simulink model "typeAsimctrl_NB_upgrade_2016b"  (R2016b)
settings: Solver=ode45  StartTime=0.0  StopTime=12.0  RelTol=1e-3  EnableMultiTasking=on
values from neighbouring files (symbols this model uses):
  gain_actIML = 2.1e-7*1.e+6*20/(2^16)/magIM(inddc)*gain_actIML    [TypeA_reconstruction.m]
  gain_actMNL = 5.1e-6*1.e+6*20/(2^16)/magMN(inddc)*gain_actMNL    [TypeA_reconstruction.m]
  gain_actTML = 1.7e-7*1.e+6*20/(2^16)/magTM(inddc)*gain_actTML    [TypeA_reconstruction.m]
  gainBFL = 0    [main.m]
  gainIPL = 0    [main.m]
  gainSCL = 1    [TypeA_reconstruction.m]
  gainSCT = 1    [TypeA_reconstruction.m]
  sys1 = sys1_exp    [check_exportvsmake.m]    (also in sumcon2mdlconst_typeA.m = sus.ss)
undefined symbols (not defined in the file or in its folder): cMat_BF, cMat_IM, cMat_MN, cMat_TM, Filt, gain_actBFGAS, gain_actBFL, gain_actBFP, gain_actBFR, gain_actBFT, gain_actBFV, gain_actBFY, gain_actF0GAS, gain_actF1GAS, gain_actF2GAS, gain_actF3GAS, gain_actIMP, gain_actIMR, gain_actIMT, gain_actIMV, gain_actIMY, gain_actIPL, gain_actIPT, gain_actIPY, gain_actMNP, gain_actMNR, gain_actMNT, gain_actMNV, gain_actMNY, gain_actTMP, gain_actTMY, gainBFP, gainBFR, gainBFT, gainBFV, gainBFY, gainBP, gainGASBF, gainGASF0, gainGASF1, gainGASF2, gainGASF3, gainIML, gainIMP, gainIMR, gainIMT, gainIMV, gainIMY, gainIPT, gainIPY, gainLOCK_IML, gainLOCK_IMP, gainLOCK_IMY, gainMNL, gainMNLOCK_L, gainMNLOCK_P, gainMNLOCK_Y, gainMNP, gainMNR, gainMNT ... (+22)
libraries: cstblocks x77, LiveParts x77
(part 2 of 3)

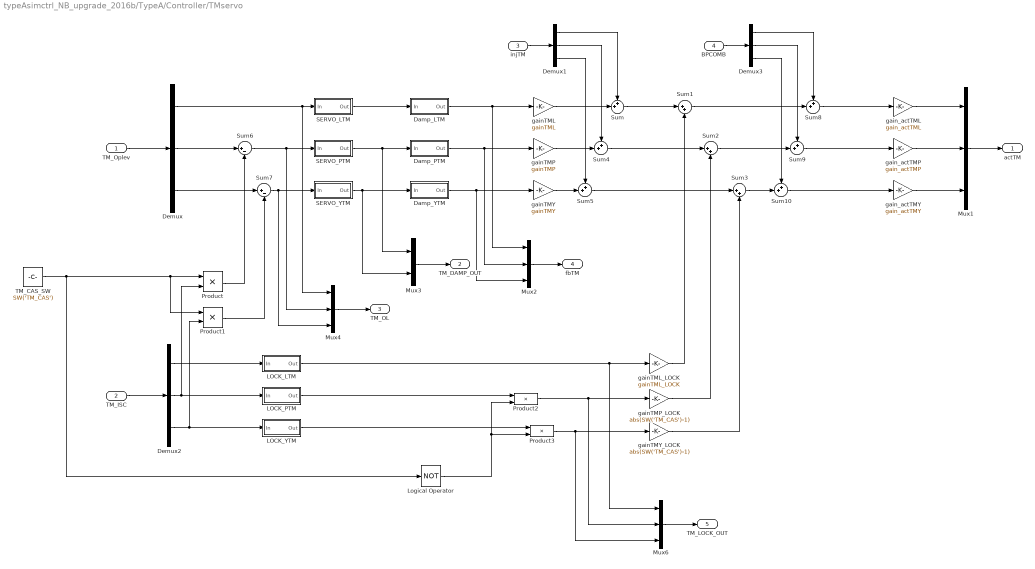
== system typeAsimctrl_NB_upgrade_2016b/TypeA/Controller/TMservo ==
  TM_Oplev : Inport
  TM_ISC : Inport  Port=2
  injTM : Inport  Port=3
  BPCOMB : Inport  Port=4
  Damp_LTM : Subsystem
  Damp_PTM : Subsystem
  Damp_YTM : Subsystem
  Demux{,1..3} (4 alike) : Demux  Outputs=3
  LOCK_LTM : Subsystem
  LOCK_PTM : Subsystem
  LOCK_YTM : Subsystem
  Logical Operator : Logic  Operator=NOT  Inputs=1  AllPortsSameDT=off  OutDataTypeStr=boolean
  Mux{1..2,4,6} (4 alike) : Mux  Inputs=3
  Mux3 : Mux  Inputs=2
  Product{,1..3} (4 alike) : Product
  SERVO_LTM : Subsystem
  SERVO_PTM : Subsystem
  SERVO_YTM : Subsystem
  Sum{,4..5,8..10} (6 alike) : Sum  Inputs=++|
  Sum1 : Sum  Inputs=|++
  Sum2 : Sum  Inputs=|++
  Sum3 : Sum  Inputs=|++
  Sum6 : Sum  Inputs=|+-
  Sum7 : Sum  Inputs=|+-
  TM_CAS_SW : Constant  Value=SW('TM_CAS')
  gainTML : Gain  Gain=gainTML
  gainTML_LOCK : Gain  Gain=gainTML_LOCK
  gainTMP : Gain  Gain=gainTMP
  gainTMP_LOCK : Gain  Gain=abs(SW('TM_CAS')-1)
  gainTMY : Gain  Gain=gainTMY
  gainTMY_LOCK : Gain  Gain=abs(SW('TM_CAS')-1)
  gain_actTML : Gain  Gain=gain_actTML
  gain_actTMP : Gain  Gain=gain_actTMP
  gain_actTMY : Gain  Gain=gain_actTMY
  actTM : Outport
  TM_DAMP_OUT : Outport  Port=2
  TM_OL : Outport  Port=3
  fbTM : Outport  Port=4
  TM_LOCK_OUT : Outport  Port=5
  wires:
  TM_Oplev/1 -> Demux/1
  gainTML/1 -> Sum/2
  injTM/1 -> Demux1/1
  Mux1/1 -> actTM/1
  Demux1/1 -> Sum/1
  gainTMP/1 -> Sum4/2
  gainTMY/1 -> Sum5/2
  gain_actTML/1 -> Mux1/1
  Demux1/2 -> Sum4/1
  Demux1/3 -> Sum5/1
  gain_actTMP/1 -> Mux1/2
  gain_actTMY/1 -> Mux1/3
  TM_ISC/1 -> Demux2/1
  SERVO_PTM/1(Out) -> Mux3/1, Damp_PTM/1(In)
  SERVO_YTM/1(Out) -> Mux3/2, Damp_YTM/1(In)
  Mux3/1 -> TM_DAMP_OUT/1
  Demux2/1 -> LOCK_LTM/1(In)
  Demux2/2 -> Product/2, LOCK_PTM/1(In)
  Demux2/3 -> Product1/2, LOCK_YTM/1(In)
  SERVO_LTM/1(Out) -> Damp_LTM/1(In)
  Sum/1 -> Sum1/1
  Sum4/1 -> Sum2/1
  Sum5/1 -> Sum3/1
  TM_CAS_SW/1 -> Logical Operator/1, Product/1, Product1/1
  Demux/2 -> Sum6/1
  Demux/3 -> Sum7/1
  Sum7/1 -> Mux4/3, SERVO_YTM/1(In)
  Product/1 -> Sum6/2
  Product1/1 -> Sum7/2
  Demux/1 -> Mux4/1, SERVO_LTM/1(In)
  Sum6/1 -> Mux4/2, SERVO_PTM/1(In)
  Mux4/1 -> TM_OL/1
  LOCK_PTM/1(Out) -> Product2/1
  Logical Operator/1 -> Product3/2, Product2/2
  LOCK_YTM/1(Out) -> Product3/1
  BPCOMB/1 -> Demux3/1
  Demux3/1 -> Sum8/1
  Demux3/2 -> Sum9/1
  Demux3/3 -> Sum10/1
  Sum1/1 -> Sum8/2
  Sum2/1 -> Sum9/2
  Sum3/1 -> Sum10/2
  Sum8/1 -> gain_actTML/1
  Sum9/1 -> gain_actTMP/1
  Sum10/1 -> gain_actTMY/1
  Damp_LTM/1(Out) -> Mux2/1, gainTML/1
  Mux2/1 -> fbTM/1
  Damp_PTM/1(Out) -> Mux2/2, gainTMP/1
  Damp_YTM/1(Out) -> Mux2/3, gainTMY/1
  Product3/1 -> Mux6/3, gainTMY_LOCK/1
  LOCK_LTM/1(Out) -> gainTML_LOCK/1, Mux6/1
  Product2/1 -> Mux6/2, gainTMP_LOCK/1
  Mux6/1 -> TM_LOCK_OUT/1
  gainTMP_LOCK/1 -> Sum2/2
  gainTML_LOCK/1 -> Sum1/2
  gainTMY_LOCK/1 -> Sum3/2

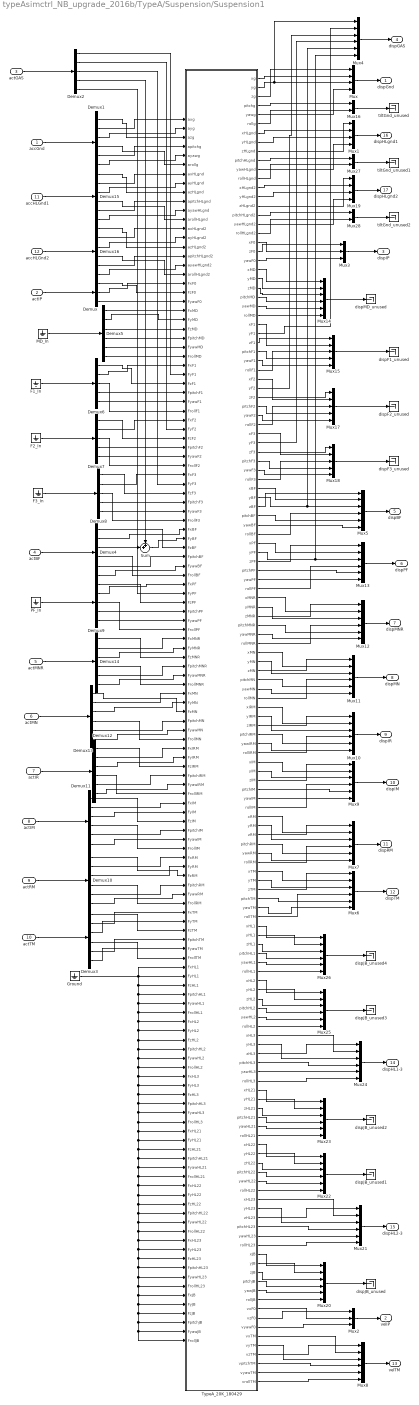
== system typeAsimctrl_NB_upgrade_2016b/TypeA/Suspension/Suspension1 ==
  accGnd : Inport
  actIP : Inport  Port=2
  actGAS : Inport  Port=3
  actBF : Inport  Port=4
  actMNR : Inport  Port=5
  actMN : Inport  Port=6
  actIR : Inport  Port=7
  actIM : Inport  Port=8
  actRM : Inport  Port=9
  actTM : Inport  Port=10
  accHLGnd1 : Inport  Port=11
  accHLGnd2 : Inport  Port=12
  Demux : Demux  Outputs=3
  Demux{1,3..5,10..16} (11 alike) : Demux  Outputs=6
  Demux{2,6..9} (5 alike) : Demux  Outputs=5
  F1_In : Ground
  F2_In : Ground
  F3_In : Ground
  Ground : Ground
  MD_In : Ground
  Mux : Mux
  Mux1 : Mux
  Mux{4..14,20..26} (18 alike) : Mux  Inputs=6
  Mux15 : Mux  Inputs=5
  Mux16 : Mux  Inputs=2
  Mux17 : Mux  Inputs=5
  Mux18 : Mux  Inputs=5
  Mux19 : Mux
  Mux2 : Mux  Inputs=3
  Mux27 : Mux  Inputs=2
  Mux28 : Mux  Inputs=2
  Mux3 : Mux  Inputs=3
  PF_In : Ground
  Sum : Sum  Inputs=++|
  TypeA_20K_180429 : Subsystem
  dispF1_unused : Terminator
  dispF2_unused : Terminator
  dispF3_unused : Terminator
  dispJB_unused{,1..4} (5 alike) : Terminator
  dispMD_unused : Terminator
  tiltGnd_unused : Terminator
  tiltGnd_unused1 : Terminator
  tiltGnd_unused2 : Terminator
  dispGnd : Outport
  velIP : Outport  Port=2
  dispIP : Outport  Port=3
  dispGAS : Outport  Port=4
  dispBF : Outport  Port=5
  dispPF : Outport  Port=6
  dispMNR : Outport  Port=7
  dispMN : Outport  Port=8
  dispIR : Outport  Port=9
  dispIM : Outport  Port=10
  dispRM : Outport  Port=11
  dispTM : Outport  Port=12
  velTM : Outport  Port=13
  dispHL1-3 : Outport  Port=14
  dispHL2-3 : Outport  Port=15
  dispHLgnd1 : Outport  Port=16
  dispHLgnd2 : Outport  Port=17
  wires:
  Mux/1 -> dispGnd/1
  Mux2/1 -> velIP/1
  Mux3/1 -> dispIP/1
  Mux4/1 -> dispGAS/1
  Mux5/1 -> dispBF/1
  Mux6/1 -> dispTM/1
  actIP/1 -> Demux/1
  accGnd/1 -> Demux1/1
  actTM/1 -> Demux3/1
  Demux4/3 -> Sum/2
  Demux2/4 -> Sum/1
  Demux2/5 -> TypeA_20K_180429/53(FyPF)
  actBF/1 -> Demux4/1
  actGAS/1 -> Demux2/1
  MD_In/1 -> Demux5/1
  Demux5/1 -> TypeA_20K_180429/22(FxMD)
  Demux5/2 -> TypeA_20K_180429/23(FyMD)
  Demux5/3 -> TypeA_20K_180429/24(FzMD)
  Demux5/4 -> TypeA_20K_180429/25(FpitchMD)
  Demux5/5 -> TypeA_20K_180429/26(FyawMD)
  Demux5/6 -> TypeA_20K_180429/27(FrollMD)
  Demux2/1 -> TypeA_20K_180429/29(FyF1)
  Demux2/2 -> TypeA_20K_180429/35(FyF2)
  Demux2/3 -> TypeA_20K_180429/41(FyF3)
  F1_In/1 -> Demux6/1
  F2_In/1 -> Demux7/1
  F3_In/1 -> Demux8/1
  Demux4/1 -> TypeA_20K_180429/48(FzBF)
  PF_In/1 -> Demux9/1
  actRM/1 -> Demux10/1
  actIM/1 -> Demux11/1
  actIR/1 -> Demux12/1
  actMN/1 -> Demux13/1
  actMNR/1 -> Demux14/1
  Demux10/5 -> TypeA_20K_180429/85(FpitchRM)
  Demux10/4 -> TypeA_20K_180429/87(FrollRM)
  Demux10/3 -> TypeA_20K_180429/83(FyRM)
  Demux10/1 -> TypeA_20K_180429/84(FzRM)
  Demux10/2 -> TypeA_20K_180429/82(FxRM)
  Demux3/3 -> TypeA_20K_180429/89(FyTM)
  Demux3/1 -> TypeA_20K_180429/90(FzTM)
  Demux3/2 -> TypeA_20K_180429/88(FxTM)
  Demux3/4 -> TypeA_20K_180429/93(FrollTM)
  Demux3/5 -> TypeA_20K_180429/91(FpitchTM)
  Demux3/6 -> TypeA_20K_180429/92(FyawTM)
  Mux7/1 -> dispRM/1
  Mux8/1 -> velTM/1
  Mux9/1 -> dispIM/1
  Mux10/1 -> dispIR/1
  Mux11/1 -> dispMN/1
  Mux12/1 -> dispMNR/1
  Mux13/1 -> dispPF/1
  Mux14/1 -> dispMD_unused/1
  Mux15/1 -> dispF1_unused/1
  Mux16/1 -> tiltGnd_unused/1
  Mux17/1 -> dispF2_unused/1
  Mux18/1 -> dispF3_unused/1
  TypeA_20K_180429/1(xg) -> Mux/2
  TypeA_20K_180429/3(zg) -> Mux/1
  TypeA_20K_180429/138(vyawF0) -> Mux2/3
  TypeA_20K_180429/19(xF0) -> Mux3/2
  TypeA_20K_180429/20(zF0) -> Mux3/1
  TypeA_20K_180429/21(yawF0) -> Mux3/3
  TypeA_20K_180429/24(zMD) -> Mux14/3
  TypeA_20K_180429/25(pitchMD) -> Mux14/4
  TypeA_20K_180429/26(yawMD) -> Mux14/5
  TypeA_20K_180429/27(rollMD) -> Mux14/6
  TypeA_20K_180429/29(yF1) -> Mux4/2
  TypeA_20K_180429/35(yF2) -> Mux4/3
  TypeA_20K_180429/41(yF3) -> Mux4/4
  TypeA_20K_180429/47(yBF) -> Mux5/3, Mux4/5
  TypeA_20K_180429/53(yPF) -> Mux13/3, Mux4/6
  TypeA_20K_180429/30(zF1) -> Mux15/1
  TypeA_20K_180429/28(xF1) -> Mux15/2
  TypeA_20K_180429/32(yawF1) -> Mux15/5
  TypeA_20K_180429/33(rollF1) -> Mux15/3
  TypeA_20K_180429/31(pitchF1) -> Mux15/4
  TypeA_20K_180429/36(zF2) -> Mux17/1
  TypeA_20K_180429/34(xF2) -> Mux17/2
  TypeA_20K_180429/39(rollF2) -> Mux17/3
  TypeA_20K_180429/38(yawF2) -> Mux17/5
  TypeA_20K_180429/37(pitchF2) -> Mux17/4
  TypeA_20K_180429/42(zF3) -> Mux18/1
  TypeA_20K_180429/40(xF3) -> Mux18/2
  TypeA_20K_180429/44(yawF3) -> Mux18/5
  TypeA_20K_180429/43(pitchF3) -> Mux18/4
  TypeA_20K_180429/45(rollF3) -> Mux18/3
  TypeA_20K_180429/49(pitchBF) -> Mux5/5
  TypeA_20K_180429/50(yawBF) -> Mux5/6
  TypeA_20K_180429/51(rollBF) -> Mux5/4
  TypeA_20K_180429/46(xBF) -> Mux5/2
  TypeA_20K_180429/48(zBF) -> Mux5/1
  TypeA_20K_180429/56(yawPF) -> Mux13/6
  TypeA_20K_180429/54(zPF) -> Mux13/1
  TypeA_20K_180429/52(xPF) -> Mux13/2
  TypeA_20K_180429/57(rollPF) -> Mux13/4
  TypeA_20K_180429/55(pitchPF) -> Mux13/5
  TypeA_20K_180429/58(xMNR) -> Mux12/2
  TypeA_20K_180429/62(yawMNR) -> Mux12/6
  TypeA_20K_180429/59(yMNR) -> Mux12/3
  TypeA_20K_180429/63(rollMNR) -> Mux12/4
  TypeA_20K_180429/60(zMNR) -> Mux12/1
  TypeA_20K_180429/61(pitchMNR) -> Mux12/5
  TypeA_20K_180429/69(rollMN) -> Mux11/4
  TypeA_20K_180429/66(zMN) -> Mux11/1
  TypeA_20K_180429/65(yMN) -> Mux11/3
  TypeA_20K_180429/64(xMN) -> Mux11/2
  TypeA_20K_180429/68(yawMN) -> Mux11/6
  TypeA_20K_180429/67(pitchMN) -> Mux11/5
  TypeA_20K_180429/73(pitchIRM) -> Mux10/5
  TypeA_20K_180429/71(yIRM) -> Mux10/3
  TypeA_20K_180429/74(yawIRM) -> Mux10/6
  TypeA_20K_180429/75(rollIRM) -> Mux10/4
  TypeA_20K_180429/70(xIRM) -> Mux10/2
  TypeA_20K_180429/72(zIRM) -> Mux10/1
  TypeA_20K_180429/78(zIM) -> Mux9/1
  TypeA_20K_180429/77(yIM) -> Mux9/3
  TypeA_20K_180429/76(xIM) -> Mux9/2
  TypeA_20K_180429/141(vzTM) -> Mux8/1
  TypeA_20K_180429/139(vxTM) -> Mux8/2
  TypeA_20K_180429/140(vyTM) -> Mux8/3
  TypeA_20K_180429/142(vpitchTM) -> Mux8/4
  TypeA_20K_180429/143(vyawTM) -> Mux8/5
  TypeA_20K_180429/144(vrollTM) -> Mux8/6
  TypeA_20K_180429/90(zTM) -> Mux6/1
  TypeA_20K_180429/88(xTM) -> Mux6/2
  TypeA_20K_180429/89(yTM) -> Mux6/3
  TypeA_20K_180429/84(zRM) -> Mux7/1
  TypeA_20K_180429/82(xRM) -> Mux7/2
  TypeA_20K_180429/83(yRM) -> Mux7/3
  TypeA_20K_180429/81(rollIM) -> Mux9/4
  TypeA_20K_180429/79(pitchIM) -> Mux9/5
  TypeA_20K_180429/80(yawIM) -> Mux9/6
  TypeA_20K_180429/87(rollRM) -> Mux7/4
  TypeA_20K_180429/85(pitchRM) -> Mux7/5
  TypeA_20K_180429/86(yawRM) -> Mux7/6
  TypeA_20K_180429/93(rollTM) -> Mux6/4
  TypeA_20K_180429/91(pitchTM) -> Mux6/5
  TypeA_20K_180429/92(yawTM) -> Mux6/6
  TypeA_20K_180429/22(xMD) -> Mux14/1
  TypeA_20K_180429/23(yMD) -> Mux14/2
  TypeA_20K_180429/136(vxF0) -> Mux2/2
  TypeA_20K_180429/137(vzF0) -> Mux2/1
  TypeA_20K_180429/2(yg) -> Mux4/1, Mux/3
  TypeA_20K_180429/5(yawg) -> Mux/4
  TypeA_20K_180429/4(pitchg) -> Mux16/1
  TypeA_20K_180429/6(rollg) -> Mux16/2
  Demux10/6 -> TypeA_20K_180429/86(FyawRM)
  Demux11/1 -> TypeA_20K_180429/78(FzIM)
  Demux11/2 -> TypeA_20K_180429/76(FxIM)
  Demux11/3 -> TypeA_20K_180429/77(FyIM)
  Demux11/4 -> TypeA_20K_180429/81(FrollIM)
  Demux11/5 -> TypeA_20K_180429/79(FpitchIM)
  Demux11/6 -> TypeA_20K_180429/80(FyawIM)
  Demux12/1 -> TypeA_20K_180429/72(FzIRM)
  Demux12/2 -> TypeA_20K_180429/70(FxIRM)
  Demux12/3 -> TypeA_20K_180429/71(FyIRM)
  Demux12/4 -> TypeA_20K_180429/75(FrollIRM)
  Demux12/5 -> TypeA_20K_180429/73(FpitchIRM)
  Demux12/6 -> TypeA_20K_180429/74(FyawIRM)
  Demux13/1 -> TypeA_20K_180429/66(FzMN)
  Demux13/2 -> TypeA_20K_180429/64(FxMN)
  Demux13/3 -> TypeA_20K_180429/65(FyMN)
  Demux13/4 -> TypeA_20K_180429/69(FrollMN)
  Demux13/5 -> TypeA_20K_180429/67(FpitchMN)
  Demux13/6 -> TypeA_20K_180429/68(FyawMN)
  Demux14/1 -> TypeA_20K_180429/60(FzMNR)
  Demux14/2 -> TypeA_20K_180429/58(FxMNR)
  Demux14/3 -> TypeA_20K_180429/59(FyMNR)
  Demux14/4 -> TypeA_20K_180429/63(FrollMNR)
  Demux14/5 -> TypeA_20K_180429/61(FpitchMNR)
  Demux14/6 -> TypeA_20K_180429/62(FyawMNR)
  Demux9/1 -> TypeA_20K_180429/54(FzPF)
  Demux9/2 -> TypeA_20K_180429/52(FxPF)
  Demux9/3 -> TypeA_20K_180429/57(FrollPF)
  Demux9/4 -> TypeA_20K_180429/55(FpitchPF)
  Demux9/5 -> TypeA_20K_180429/56(FyawPF)
  Demux4/2 -> TypeA_20K_180429/46(FxBF)
  Sum/1 -> TypeA_20K_180429/47(FyBF)
  Demux4/4 -> TypeA_20K_180429/51(FrollBF)
  Demux4/5 -> TypeA_20K_180429/49(FpitchBF)
  Demux4/6 -> TypeA_20K_180429/50(FyawBF)
  Demux8/1 -> TypeA_20K_180429/42(FzF3)
  Demux8/2 -> TypeA_20K_180429/40(FxF3)
  Demux8/3 -> TypeA_20K_180429/45(FrollF3)
  Demux8/4 -> TypeA_20K_180429/43(FpitchF3)
  Demux8/5 -> TypeA_20K_180429/44(FyawF3)
  Demux7/1 -> TypeA_20K_180429/36(FzF2)
  Demux7/2 -> TypeA_20K_180429/34(FxF2)
  Demux7/3 -> TypeA_20K_180429/39(FrollF2)
  Demux7/4 -> TypeA_20K_180429/37(FpitchF2)
  Demux7/5 -> TypeA_20K_180429/38(FyawF2)
  Demux6/1 -> TypeA_20K_180429/30(FzF1)
  Demux6/2 -> TypeA_20K_180429/28(FxF1)
  Demux6/3 -> TypeA_20K_180429/33(FrollF1)
  Demux6/4 -> TypeA_20K_180429/31(FpitchF1)
  Demux6/5 -> TypeA_20K_180429/32(FyawF1)
  Demux/1 -> TypeA_20K_180429/20(FzF0)
  Demux/2 -> TypeA_20K_180429/19(FxF0)
  Demux/3 -> TypeA_20K_180429/21(FyawF0)
  Demux1/1 -> TypeA_20K_180429/3(azg)
  Demux1/2 -> TypeA_20K_180429/1(axg)
  Demux1/3 -> TypeA_20K_180429/2(ayg)
  Demux1/4 -> TypeA_20K_180429/6(arollg)
  Demux1/5 -> TypeA_20K_180429/4(apitchg)
  Demux1/6 -> TypeA_20K_180429/5(ayawg)
  TypeA_20K_180429/132(zJB) -> Mux20/3
  TypeA_20K_180429/131(yJB) -> Mux20/2
  TypeA_20K_180429/134(yawJB) -> Mux20/5
  TypeA_20K_180429/135(rollJB) -> Mux20/6
  TypeA_20K_180429/130(xJB) -> Mux20/1
  TypeA_20K_180429/133(pitchJB) -> Mux20/4
  Mux20/1 -> dispJB_unused/1
  TypeA_20K_180429/128(yawHL23) -> Mux21/5
  TypeA_20K_180429/129(rollHL23) -> Mux21/6
  TypeA_20K_180429/124(xHL23) -> Mux21/2
  TypeA_20K_180429/127(pitchHL23) -> Mux21/4
  TypeA_20K_180429/125(yHL23) -> Mux21/3
  TypeA_20K_180429/126(zHL23) -> Mux21/1
  Mux21/1 -> dispHL2-3/1
  TypeA_20K_180429/122(yawHL22) -> Mux22/5
  TypeA_20K_180429/120(zHL22) -> Mux22/3
  TypeA_20K_180429/119(yHL22) -> Mux22/2
  TypeA_20K_180429/121(pitchHL22) -> Mux22/4
  TypeA_20K_180429/123(rollHL22) -> Mux22/6
  TypeA_20K_180429/118(xHL22) -> Mux22/1
  Mux22/1 -> dispJB_unused1/1
  TypeA_20K_180429/116(yawHL21) -> Mux23/5
  TypeA_20K_180429/114(zHL21) -> Mux23/3
  TypeA_20K_180429/113(yHL21) -> Mux23/2
  TypeA_20K_180429/115(pitchHL21) -> Mux23/4
  TypeA_20K_180429/117(rollHL21) -> Mux23/6
  TypeA_20K_180429/112(xHL21) -> Mux23/1
  Mux23/1 -> dispJB_unused2/1
  TypeA_20K_180429/110(yawHL3) -> Mux24/5
  TypeA_20K_180429/111(rollHL3) -> Mux24/6
  TypeA_20K_180429/109(pitchHL3) -> Mux24/4
  TypeA_20K_180429/107(yHL3) -> Mux24/3
  TypeA_20K_180429/108(zHL3) -> Mux24/1
  TypeA_20K_180429/106(xHL3) -> Mux24/2
  Mux24/1 -> dispHL1-3/1
  TypeA_20K_180429/104(yawHL2) -> Mux25/5
  Mux25/1 -> dispJB_unused3/1
  TypeA_20K_180429/102(zHL2) -> Mux25/3
  TypeA_20K_180429/103(pitchHL2) -> Mux25/4
  TypeA_20K_180429/105(rollHL2) -> Mux25/6
  TypeA_20K_180429/100(xHL2) -> Mux25/1
  TypeA_20K_180429/101(yHL2) -> Mux25/2
  TypeA_20K_180429/98(yawHL1) -> Mux26/5
  Mux26/1 -> dispJB_unused4/1
  TypeA_20K_180429/96(zHL1) -> Mux26/3
  TypeA_20K_180429/97(pitchHL1) -> Mux26/4
  TypeA_20K_180429/99(rollHL1) -> Mux26/6
  TypeA_20K_180429/94(xHL1) -> Mux26/1
  TypeA_20K_180429/95(yHL1) -> Mux26/2
  TypeA_20K_180429/9(zHLgnd) -> Mux1/1
  TypeA_20K_180429/7(xHLgnd) -> Mux1/2
  TypeA_20K_180429/8(yHLgnd) -> Mux1/3
  TypeA_20K_180429/11(yawHLgnd) -> Mux1/4
  Mux1/1 -> dispHLgnd1/1
  Mux19/1 -> dispHLgnd2/1
  TypeA_20K_180429/14(yHLgnd2) -> Mux19/3
  TypeA_20K_180429/15(zHLgnd2) -> Mux19/1
  TypeA_20K_180429/13(xHLgnd2) -> Mux19/2
  TypeA_20K_180429/17(yawHLgnd2) -> Mux19/4
  TypeA_20K_180429/10(pitchHLgnd) -> Mux27/1
  TypeA_20K_180429/12(rollHLgnd) -> Mux27/2
  Mux27/1 -> tiltGnd_unused1/1
  TypeA_20K_180429/16(pitchHLgnd2) -> Mux28/1
  TypeA_20K_180429/18(rollHLgnd2) -> Mux28/2
  Mux28/1 -> tiltGnd_unused2/1
  Ground/1 -> TypeA_20K_180429/96(FzHL1), TypeA_20K_180429/97(FpitchHL1), TypeA_20K_180429/98(FyawHL1), TypeA_20K_180429/99(FrollHL1), TypeA_20K_180429/100(FxHL2), TypeA_20K_180429/101(FyHL2), TypeA_20K_180429/102(FzHL2), TypeA_20K_180429/103(FpitchHL2), TypeA_20K_180429/104(FyawHL2), TypeA_20K_180429/105(FrollHL2), TypeA_20K_180429/106(FxHL3), TypeA_20K_180429/107(FyHL3), TypeA_20K_180429/108(FzHL3), TypeA_20K_180429/109(FpitchHL3), TypeA_20K_180429/110(FyawHL3), TypeA_20K_180429/111(FrollHL3), TypeA_20K_180429/112(FxHL21), TypeA_20K_180429/113(FyHL21), TypeA_20K_180429/114(FzHL21), TypeA_20K_180429/115(FpitchHL21), TypeA_20K_180429/116(FyawHL21), TypeA_20K_180429/117(FrollHL21), TypeA_20K_180429/118(FxHL22), TypeA_20K_180429/119(FyHL22), TypeA_20K_180429/120(FzHL22), TypeA_20K_180429/121(FpitchHL22), TypeA_20K_180429/122(FyawHL22), TypeA_20K_180429/123(FrollHL22), TypeA_20K_180429/124(FxHL23), TypeA_20K_180429/125(FyHL23), TypeA_20K_180429/126(FzHL23), TypeA_20K_180429/127(FpitchHL23), TypeA_20K_180429/128(FyawHL23), TypeA_20K_180429/129(FrollHL23), TypeA_20K_180429/130(FxJB), TypeA_20K_180429/131(FyJB), TypeA_20K_180429/132(FzJB), TypeA_20K_180429/133(FpitchJB), TypeA_20K_180429/134(FyawJB), TypeA_20K_180429/135(FrollJB), TypeA_20K_180429/95(FyHL1), TypeA_20K_180429/94(FxHL1)
  Demux15/4 -> TypeA_20K_180429/12(arollHLgnd)
  Demux15/5 -> TypeA_20K_180429/10(apitchHLgnd)
  Demux15/1 -> TypeA_20K_180429/9(azHLgnd)
  Demux15/2 -> TypeA_20K_180429/7(axHLgnd)
  Demux15/6 -> TypeA_20K_180429/11(ayawHLgnd)
  accHLGnd1/1 -> Demux15/1
  Demux15/3 -> TypeA_20K_180429/8(ayHLgnd)
  Demux16/4 -> TypeA_20K_180429/18(arollHLgnd2)
  Demux16/5 -> TypeA_20K_180429/16(apitchHLgnd2)
  Demux16/1 -> TypeA_20K_180429/15(azHLgnd2)
  Demux16/2 -> TypeA_20K_180429/13(axHLgnd2)
  Demux16/6 -> TypeA_20K_180429/17(ayawHLgnd2)
  accHLGnd2/1 -> Demux16/1
  Demux16/3 -> TypeA_20K_180429/14(ayHLgnd2)

== system typeAsimctrl_NB_upgrade_2016b/TypeA/Suspension/aMatrix_BF ==
  aMat_in : Inport
  cMat_BF : Constant  Value=cMat_BF  VectorParams1D=off
  coupling_BF : Product  Multiplication=Matrix(*)
  actBF : Outport
  wires:
  coupling_BF/1 -> actBF/1
  aMat_in/1 -> coupling_BF/2
  cMat_BF/1 -> coupling_BF/1

== system typeAsimctrl_NB_upgrade_2016b/TypeA/Suspension/aMatrix_GAS ==
  aMat_in : Inport
  Add{1..4} (4 alike) : Sum  Inputs=+-
  Demux4 : Demux  Outputs=5
  Mux3 : Mux  Inputs=5
  actGAS : Outport
  wires:
  aMat_in/1 -> Demux4/1
  Mux3/1 -> actGAS/1
  Add1/1 -> Mux3/1
  Add2/1 -> Mux3/2
  Demux4/3 -> Add3/1, Add2/2
  Demux4/2 -> Add1/2, Add2/1
  Demux4/1 -> Add1/1
  Demux4/5 -> Mux3/5, Add4/2
  Add4/1 -> Mux3/4
  Add3/1 -> Mux3/3
  Demux4/4 -> Add3/2, Add4/1

== system typeAsimctrl_NB_upgrade_2016b/TypeA/Suspension/aMatrix_IM ==
  aMat_in : Inport
  Gain : Gain  Gain=-1
  cMat_IM : Constant  Value=cMat_IM  VectorParams1D=off
  coupling_IM : Product  Multiplication=Matrix(*)
  actIR : Outport
  actIM : Outport  Port=2
  wires:
  coupling_IM/1 -> actIM/1, Gain/1
  aMat_in/1 -> coupling_IM/2
  cMat_IM/1 -> coupling_IM/1
  Gain/1 -> actIR/1

== system typeAsimctrl_NB_upgrade_2016b/TypeA/Suspension/aMatrix_MN ==
  aMat_in : Inport
  Gain : Gain  Gain=-1
  cMat_MN : Constant  Value=cMat_MN  VectorParams1D=off
  coupling_MN : Product  Multiplication=Matrix(*)
  actMNR : Outport
  actMN : Outport  Port=2
  wires:
  coupling_MN/1 -> actMN/1, Gain/1
  aMat_in/1 -> coupling_MN/2
  cMat_MN/1 -> coupling_MN/1
  Gain/1 -> actMNR/1

== system typeAsimctrl_NB_upgrade_2016b/TypeA/Suspension/aMatrix_TM ==
  aMat_in : Inport
  Demux : Demux  Outputs=3
  Demux1 : Demux  Outputs=3
  Gain : Gain  Gain=-1
  Ground{,1..5} (6 alike) : Ground
  Mux : Mux  Inputs=6
  Mux1 : Mux  Inputs=6
  cMat_TM : Constant  Value=cMat_TM  VectorParams1D=off
  coupling_TM : Product  Multiplication=Matrix(*)
  actRM : Outport
  actTM : Outport  Port=2
  wires:
  coupling_TM/1 -> Demux1/1, Gain/1
  aMat_in/1 -> coupling_TM/2  "3DoF"
  cMat_TM/1 -> coupling_TM/1
  Gain/1 -> Demux/1
  Demux/1 -> Mux/1
  Demux/2 -> Mux/5
  Demux/3 -> Mux/6
  Demux1/1 -> Mux1/1
  Demux1/3 -> Mux1/6
  Demux1/2 -> Mux1/5
  Ground/1 -> Mux/2
  Ground1/1 -> Mux/3
  Ground2/1 -> Mux/4
  Ground4/1 -> Mux1/3
  Ground3/1 -> Mux1/2
  Ground5/1 -> Mux1/4
  Mux/1 -> actRM/1  "6DoF"
  Mux1/1 -> actTM/1  "6DoF"

== system typeAsimctrl_NB_upgrade_2016b/TypeA/Suspension/sMatrix_BF_LVDT ==
  dispGnd : Inport
  dispBF : Inport  Port=2
  Add2 : Sum  Inputs=-+
  Demux : Demux
  Ground : Ground
  Ground1 : Ground
  Mux : Mux  Inputs=6
  BF_LVDT : Outport
  wires:
  Add2/1 -> BF_LVDT/1  "6DoF"
  dispBF/1 -> Add2/2  "6DoF"
  dispGnd/1 -> Demux/1  "4DoF"
  Demux/1 -> Mux/1  "L"
  Demux/2 -> Mux/2  "T"
  Demux/3 -> Mux/3  "V"
  Demux/4 -> Mux/6  "Y"
  Ground/1 -> Mux/4  "R"
  Ground1/1 -> Mux/5  "P"
  Mux/1 -> Add2/1

== system typeAsimctrl_NB_upgrade_2016b/TypeA/Suspension/sMatrix_GAS_LVDT ==
  dispGAS : Inport
  Add{1..5} (5 alike) : Sum  Inputs=-+
  Demux4 : Demux  Outputs=6
  Mux3 : Mux  Inputs=5
  GAS_LVDT : Outport
  wires:
  dispGAS/1 -> Demux4/1
  Demux4/1 -> Add2/1  "VGnd = IPV"
  Demux4/2 -> Add1/1, Add2/2  "VF1"
  Demux4/3 -> Add1/2, Add3/1  "VF2"
  Demux4/4 -> Add4/1, Add3/2  "VF3"
  Add2/1 -> Mux3/1  "GASF0"
  Add1/1 -> Mux3/2  "GASF1"
  Add3/1 -> Mux3/3  "GASF2"
  Mux3/1 -> GAS_LVDT/1
  Demux4/5 -> Add5/1, Add4/2  "VBF"
  Demux4/6 -> Add5/2  "VPF"
  Add4/1 -> Mux3/4  "GASF3"
  Add5/1 -> Mux3/5  "GASBF"

== system typeAsimctrl_NB_upgrade_2016b/TypeA/Suspension/sMatrix_IM_PS ==
  dispIR : Inport
  dispIM : Inport  Port=2
  Add2 : Sum  Inputs=-+
  IM_PS : Outport
  wires:
  Add2/1 -> IM_PS/1
  dispIM/1 -> Add2/2
  dispIR/1 -> Add2/1

== system typeAsimctrl_NB_upgrade_2016b/TypeA/Suspension/sMatrix_IP_LVDT ==
  dispGnd : Inport
  dispIP : Inport  Port=2
  Add2 : Sum  Inputs=-+
  Demux : Demux
  Mux : Mux  Inputs=3
  Terminator : Terminator
  IP_LVDT : Outport
  wires:
  Add2/1 -> IP_LVDT/1
  dispIP/1 -> Add2/2
  dispGnd/1 -> Demux/1
  Demux/1 -> Mux/1  "L"
  Demux/2 -> Mux/2  "T"
  Demux/4 -> Mux/3  "Y"
  Demux/3 -> Terminator/1  "V"
  Mux/1 -> Add2/1

== system typeAsimctrl_NB_upgrade_2016b/TypeA/Suspension/sMatrix_MN_OpLev ==
  dispMN : Inport
  dispGND : Inport  Port=2
  Demux : Demux  Outputs=6
  Demux1 : Demux
  Mux : Mux  Inputs=6
  Sum : Sum  Inputs=-+|
  Sum1 : Sum  Inputs=-+|
  Sum2 : Sum  Inputs=-+|
  Terminator : Terminator
  MN_OpLev : Outport
  wires:
  dispMN/1 -> Demux/1
  dispGND/1 -> Demux1/1
  Demux/1 -> Sum/2
  Demux1/1 -> Sum/1
  Demux1/2 -> Sum1/1
  Demux/2 -> Sum1/2
  Demux/3 -> Sum2/2
  Demux1/3 -> Sum2/1
  Demux1/4 -> Terminator/1
  Sum/1 -> Mux/1
  Sum1/1 -> Mux/2
  Sum2/1 -> Mux/3
  Demux/4 -> Mux/4
  Demux/5 -> Mux/5
  Demux/6 -> Mux/6
  Mux/1 -> MN_OpLev/1

== system typeAsimctrl_NB_upgrade_2016b/TypeA/Suspension/sMatrix_MN_PS ==
  dispMNR : Inport
  dispMN : Inport  Port=2
  Add2 : Sum  Inputs=-+
  MN_PS : Outport
  wires:
  Add2/1 -> MN_PS/1
  dispMN/1 -> Add2/2
  dispMNR/1 -> Add2/1

== system typeAsimctrl_NB_upgrade_2016b/TypeA/Suspension/sMatrix_PF_OpLev ==
  dispPF : Inport
  dispGND : Inport  Port=2
  Demux : Demux
  Demux4 : Demux  Outputs=6
  Mux3 : Mux  Inputs=3
  Sum : Sum  Inputs=-+|
  Terminator : Terminator
  Terminator1 : Terminator
  Terminator2 : Terminator
  dispRPF : Terminator
  dispTPF : Terminator
  dispVPF : Terminator
  OpLev_PF : Outport
  wires:
  dispPF/1 -> Demux4/1
  Mux3/1 -> OpLev_PF/1
  Demux4/2 -> dispTPF/1
  Demux4/3 -> dispVPF/1
  Demux4/5 -> Mux3/2
  Demux4/6 -> Mux3/3
  Demux4/4 -> dispRPF/1
  Demux4/1 -> Sum/2
  Sum/1 -> Mux3/1
  dispGND/1 -> Demux/1
  Demux/1 -> Sum/1
  Demux/2 -> Terminator/1
  Demux/3 -> Terminator1/1
  Demux/4 -> Terminator2/1

== system typeAsimctrl_NB_upgrade_2016b/TypeA/Suspension/sMatrix_TM_OpLev ==
  dispTM : Inport
  dispGND : Inport  Port=2
  Add : Sum  Inputs=-+
  Demux : Demux
  Demux4 : Demux  Outputs=6
  Mux3 : Mux  Inputs=3
  dispTMR : Terminator
  dispTMT{,1..3} (4 alike) : Terminator
  dispTMV : Terminator
  TM_OpLev : Outport
  wires:
  dispTM/1 -> Demux4/1
  Mux3/1 -> TM_OpLev/1
  Demux4/2 -> dispTMT/1
  Demux4/3 -> dispTMV/1
  Demux4/4 -> dispTMR/1
  Demux4/5 -> Mux3/2
  Demux4/6 -> Mux3/3
  Demux/1 -> Add/1
  dispGND/1 -> Demux/1
  Demux/2 -> dispTMT1/1
  Demux/3 -> dispTMT2/1
  Demux/4 -> dispTMT3/1
  Demux4/1 -> Add/2
  Add/1 -> Mux3/1

== system typeAsimctrl_NB_upgrade_2016b/TypeA/Suspension/sMatrix_TM_PS ==
  dispRM : Inport
  dispTM : Inport  Port=2
  Add2 : Sum  Inputs=-+
  Demux : Demux  Outputs=6
  Demux1 : Demux  Outputs=6
  Mux : Mux  Inputs=3
  Mux1 : Mux  Inputs=3
  Terminator{,1..5} (6 alike) : Terminator
  TM_PS : Outport
  wires:
  Add2/1 -> TM_PS/1  "(L, P, Y)"
  dispRM/1 -> Demux/1
  dispTM/1 -> Demux1/1
  Demux/1 -> Mux/1  "L"
  Demux/5 -> Mux/2  "P"
  Demux/6 -> Mux/3  "Y"
  Demux1/1 -> Mux1/1  "L"
  Demux1/5 -> Mux1/2  "P"
  Demux1/6 -> Mux1/3  "Y"
  Mux/1 -> Add2/1
  Mux1/1 -> Add2/2
  Demux/2 -> Terminator/1  "T"
  Demux/4 -> Terminator2/1  "R"
  Demux/3 -> Terminator1/1  "V"
  Demux1/4 -> Terminator5/1  "R"
  Demux1/2 -> Terminator3/1  "T"
  Demux1/3 -> Terminator4/1  "V"

== system typeAsimctrl_NB_upgrade_2016b/TypeA/Controller/BFservo/Servo_LBF ==
  In : Inport
  BF_DAMP_L : cstblocks/LTI System  sys=Filt('BF_DAMP_L')  IC=[]
  K1:VIS-OPTIC_BF_DAMP_L : LiveParts/LiveFilter  Tag=LiveFilter
      settings: AttributesFormatString=%<Tag>
  Out : Outport
  wires:
  In/1 -> BF_DAMP_L/1
  BF_DAMP_L/1 -> Out/1

== system typeAsimctrl_NB_upgrade_2016b/TypeA/Controller/BFservo/Servo_PBF ==
  In : Inport
  BF_DAMP_P : cstblocks/LTI System  sys=Filt('BF_DAMP_P')  IC=[]
  K1:VIS-OPTIC_BF_DAMP_P : LiveParts/LiveFilter  Tag=LiveFilter
      settings: AttributesFormatString=%<Tag>
  Out : Outport
  wires:
  In/1 -> BF_DAMP_P/1
  BF_DAMP_P/1 -> Out/1

== system typeAsimctrl_NB_upgrade_2016b/TypeA/Controller/BFservo/Servo_RBF ==
  In : Inport
  BF_DAMP_R : cstblocks/LTI System  sys=Filt('BF_DAMP_R')  IC=[]
  K1:VIS-OPTIC_BF_DAMP_R : LiveParts/LiveFilter  Tag=LiveFilter
      settings: AttributesFormatString=%<Tag>
  Out : Outport
  wires:
  In/1 -> BF_DAMP_R/1
  BF_DAMP_R/1 -> Out/1

== system typeAsimctrl_NB_upgrade_2016b/TypeA/Controller/BFservo/Servo_TBF ==
  In : Inport
  BF_DAMP_T : cstblocks/LTI System  sys=Filt('BF_DAMP_T')  IC=[]
  K1:VIS-OPTIC_BF_DAMP_T : LiveParts/LiveFilter  Tag=LiveFilter
      settings: AttributesFormatString=%<Tag>
  Out : Outport
  wires:
  In/1 -> BF_DAMP_T/1
  BF_DAMP_T/1 -> Out/1

== system typeAsimctrl_NB_upgrade_2016b/TypeA/Controller/BFservo/Servo_VBF ==
  In : Inport
  BF_DAMP_V : cstblocks/LTI System  sys=Filt('BF_DAMP_V')  IC=[]
  K1:VIS-OPTIC_BF_DAMP_V : LiveParts/LiveFilter  Tag=LiveFilter
      settings: AttributesFormatString=%<Tag>
  Out : Outport
  wires:
  In/1 -> BF_DAMP_V/1
  BF_DAMP_V/1 -> Out/1

== system typeAsimctrl_NB_upgrade_2016b/TypeA/Controller/BFservo/Servo_YBF ==
  In : Inport
  BF_DAMP_Y : cstblocks/LTI System  sys=Filt('BF_DAMP_Y')  IC=[]
  K1:VIS-OPTIC_BF_DAMP_Y : LiveParts/LiveFilter  Tag=LiveFilter
      settings: AttributesFormatString=%<Tag>
  Out : Outport
  wires:
  In/1 -> BF_DAMP_Y/1
  BF_DAMP_Y/1 -> Out/1

== system typeAsimctrl_NB_upgrade_2016b/TypeA/Controller/BPcomb/OLSERVO_20 ==
  In : Inport
  K1:VIS-OPTIC_PAY_OLSERVO_DAMP_P20 : LiveParts/LiveFilter  Tag=LiveFilter
      settings: AttributesFormatString=%<Tag>
  PAY_OLSERVO_DAMP_P20 : cstblocks/LTI System  sys=Filt('PAY_OLSERVO_DAMP_P20')  IC=[]
  Out : Outport
  wires:
  In/1 -> PAY_OLSERVO_DAMP_P20/1
  PAY_OLSERVO_DAMP_P20/1 -> Out/1

== system typeAsimctrl_NB_upgrade_2016b/TypeA/Controller/BPcomb/OLSERVO_22 ==
  In : Inport
  K1:VIS-OPTIC_PAY_OLSERVO_DAMP_P22 : LiveParts/LiveFilter  Tag=LiveFilter
      settings: AttributesFormatString=%<Tag>
  PAY_OLSERVO_DAMP_P22 : cstblocks/LTI System  sys=Filt('PAY_OLSERVO_DAMP_P22')  IC=[]
  Out : Outport
  wires:
  In/1 -> PAY_OLSERVO_DAMP_P22/1
  PAY_OLSERVO_DAMP_P22/1 -> Out/1

== system typeAsimctrl_NB_upgrade_2016b/TypeA/Controller/BPcomb/OLSERVO_P01 ==
  In : Inport
  K1:VIS-OPTIC_PAY_OLSERVO_DAMP_P01 : LiveParts/LiveFilter  Tag=LiveFilter
      settings: AttributesFormatString=%<Tag>
  PAY_OLSERVO_DAMP_P01 : cstblocks/LTI System  sys=Filt('PAY_OLSERVO_DAMP_P01')  IC=[]
  Out : Outport
  wires:
  In/1 -> PAY_OLSERVO_DAMP_P01/1
  PAY_OLSERVO_DAMP_P01/1 -> Out/1

== system typeAsimctrl_NB_upgrade_2016b/TypeA/Controller/BPcomb/OLSERVO_P02 ==
  In : Inport
  K1:VIS-OPTIC_PAY_OLSERVO_DAMP_P02 : LiveParts/LiveFilter  Tag=LiveFilter
      settings: AttributesFormatString=%<Tag>
  PAY_OLSERVO_DAMP_P02 : cstblocks/LTI System  sys=Filt('PAY_OLSERVO_DAMP_P02')  IC=[]
  Out : Outport
  wires:
  In/1 -> PAY_OLSERVO_DAMP_P02/1
  PAY_OLSERVO_DAMP_P02/1 -> Out/1

== system typeAsimctrl_NB_upgrade_2016b/TypeA/Controller/BPcomb/OLSERVO_P03 ==
  In : Inport
  K1:VIS-OPTIC_PAY_OLSERVO_DAMP_P03 : LiveParts/LiveFilter  Tag=LiveFilter
      settings: AttributesFormatString=%<Tag>
  PAY_OLSERVO_DAMP_P03 : cstblocks/LTI System  sys=Filt('PAY_OLSERVO_DAMP_P03')  IC=[]
  Out : Outport
  wires:
  In/1 -> PAY_OLSERVO_DAMP_P03/1
  PAY_OLSERVO_DAMP_P03/1 -> Out/1

== system typeAsimctrl_NB_upgrade_2016b/TypeA/Controller/BPcomb/OLSERVO_P04 ==
  In : Inport
  K1:VIS-OPTIC_PAY_OLSERVO_DAMP_P04 : LiveParts/LiveFilter  Tag=LiveFilter
      settings: AttributesFormatString=%<Tag>
  PAY_OLSERVO_DAMP_P04 : cstblocks/LTI System  sys=Filt('PAY_OLSERVO_DAMP_P04')  IC=[]
  Out : Outport
  wires:
  In/1 -> PAY_OLSERVO_DAMP_P04/1
  PAY_OLSERVO_DAMP_P04/1 -> Out/1

== system typeAsimctrl_NB_upgrade_2016b/TypeA/Controller/BPcomb/OLSERVO_P05 ==
  In : Inport
  K1:VIS-OPTIC_PAY_OLSERVO_DAMP_P05 : LiveParts/LiveFilter  Tag=LiveFilter
      settings: AttributesFormatString=%<Tag>
  PAY_OLSERVO_DAMP_P05 : cstblocks/LTI System  sys=Filt('PAY_OLSERVO_DAMP_P05')  IC=[]
  Out : Outport
  wires:
  In/1 -> PAY_OLSERVO_DAMP_P05/1
  PAY_OLSERVO_DAMP_P05/1 -> Out/1

== system typeAsimctrl_NB_upgrade_2016b/TypeA/Controller/BPcomb/OLSERVO_P06 ==
  In : Inport
  K1:VIS-OPTIC_PAY_OLSERVO_DAMP_P06 : LiveParts/LiveFilter  Tag=LiveFilter
      settings: AttributesFormatString=%<Tag>
  PAY_OLSERVO_DAMP_P06 : cstblocks/LTI System  sys=Filt('PAY_OLSERVO_DAMP_P06')  IC=[]
  Out : Outport
  wires:
  In/1 -> PAY_OLSERVO_DAMP_P06/1
  PAY_OLSERVO_DAMP_P06/1 -> Out/1

== system typeAsimctrl_NB_upgrade_2016b/TypeA/Controller/BPcomb/OLSERVO_P07 ==
  In : Inport
  K1:VIS-OPTIC_PAY_OLSERVO_DAMP_P07 : LiveParts/LiveFilter  Tag=LiveFilter
      settings: AttributesFormatString=%<Tag>
  PAY_OLSERVO_DAMP_P07 : cstblocks/LTI System  sys=Filt('PAY_OLSERVO_DAMP_P07')  IC=[]
  Out : Outport
  wires:
  In/1 -> PAY_OLSERVO_DAMP_P07/1
  PAY_OLSERVO_DAMP_P07/1 -> Out/1

== system typeAsimctrl_NB_upgrade_2016b/TypeA/Controller/BPcomb/OLSERVO_P08 ==
  In : Inport
  K1:VIS-OPTIC_PAY_OLSERVO_DAMP_P08 : LiveParts/LiveFilter  Tag=LiveFilter
      settings: AttributesFormatString=%<Tag>
  PAY_OLSERVO_DAMP_P08 : cstblocks/LTI System  sys=Filt('PAY_OLSERVO_DAMP_P08')  IC=[]
  Out : Outport
  wires:
  In/1 -> PAY_OLSERVO_DAMP_P08/1
  PAY_OLSERVO_DAMP_P08/1 -> Out/1

== system typeAsimctrl_NB_upgrade_2016b/TypeA/Controller/BPcomb/OLSERVO_P09 ==
  In : Inport
  K1:VIS-OPTIC_PAY_OLSERVO_DAMP_P09 : LiveParts/LiveFilter  Tag=LiveFilter
      settings: AttributesFormatString=%<Tag>
  PAY_OLSERVO_DAMP_P09 : cstblocks/LTI System  sys=Filt('PAY_OLSERVO_DAMP_P09')  IC=[]
  Out : Outport
  wires:
  In/1 -> PAY_OLSERVO_DAMP_P09/1
  PAY_OLSERVO_DAMP_P09/1 -> Out/1

== system typeAsimctrl_NB_upgrade_2016b/TypeA/Controller/BPcomb/OLSERVO_P10 ==
  In : Inport
  K1:VIS-OPTIC_PAY_OLSERVO_DAMP_P10 : LiveParts/LiveFilter  Tag=LiveFilter
      settings: AttributesFormatString=%<Tag>
  PAY_OLSERVO_DAMP_P10 : cstblocks/LTI System  sys=Filt('PAY_OLSERVO_DAMP_P10')  IC=[]
  Out : Outport
  wires:
  In/1 -> PAY_OLSERVO_DAMP_P10/1
  PAY_OLSERVO_DAMP_P10/1 -> Out/1

== system typeAsimctrl_NB_upgrade_2016b/TypeA/Controller/BPcomb/OLSERVO_P11 ==
  In : Inport
  K1:VIS-OPTIC_PAY_OLSERVO_DAMP_P11 : LiveParts/LiveFilter  Tag=LiveFilter
      settings: AttributesFormatString=%<Tag>
  PAY_OLSERVO_DAMP_P11 : cstblocks/LTI System  sys=Filt('PAY_OLSERVO_DAMP_P11')  IC=[]
  Out : Outport
  wires:
  In/1 -> PAY_OLSERVO_DAMP_P11/1
  PAY_OLSERVO_DAMP_P11/1 -> Out/1

== system typeAsimctrl_NB_upgrade_2016b/TypeA/Controller/BPcomb/OLSERVO_P12 ==
  In : Inport
  K1:VIS-OPTIC_PAY_OLSERVO_DAMP_P12 : LiveParts/LiveFilter  Tag=LiveFilter
      settings: AttributesFormatString=%<Tag>
  PAY_OLSERVO_DAMP_P12 : cstblocks/LTI System  sys=Filt('PAY_OLSERVO_DAMP_P12')  IC=[]
  Out : Outport
  wires:
  In/1 -> PAY_OLSERVO_DAMP_P12/1
  PAY_OLSERVO_DAMP_P12/1 -> Out/1

== system typeAsimctrl_NB_upgrade_2016b/TypeA/Controller/BPcomb/OLSERVO_P13 ==
  In : Inport
  K1:VIS-OPTIC_PAY_OLSERVO_DAMP_P13 : LiveParts/LiveFilter  Tag=LiveFilter
      settings: AttributesFormatString=%<Tag>
  PAY_OLSERVO_DAMP_P13 : cstblocks/LTI System  sys=Filt('PAY_OLSERVO_DAMP_P13')  IC=[]
  Out : Outport
  wires:
  In/1 -> PAY_OLSERVO_DAMP_P13/1
  PAY_OLSERVO_DAMP_P13/1 -> Out/1

== system typeAsimctrl_NB_upgrade_2016b/TypeA/Controller/BPcomb/OLSERVO_P14 ==
  In : Inport
  K1:VIS-OPTIC_PAY_OLSERVO_DAMP_P14 : LiveParts/LiveFilter  Tag=LiveFilter
      settings: AttributesFormatString=%<Tag>
  PAY_OLSERVO_DAMP_P14 : cstblocks/LTI System  sys=Filt('PAY_OLSERVO_DAMP_P14')  IC=[]
  Out : Outport
  wires:
  In/1 -> PAY_OLSERVO_DAMP_P14/1
  PAY_OLSERVO_DAMP_P14/1 -> Out/1

== system typeAsimctrl_NB_upgrade_2016b/TypeA/Controller/BPcomb/OLSERVO_P15 ==
  In : Inport
  K1:VIS-OPTIC_PAY_OLSERVO_DAMP_P15 : LiveParts/LiveFilter  Tag=LiveFilter
      settings: AttributesFormatString=%<Tag>
  PAY_OLSERVO_DAMP_P15 : cstblocks/LTI System  sys=Filt('PAY_OLSERVO_DAMP_P15')  IC=[]
  Out : Outport
  wires:
  In/1 -> PAY_OLSERVO_DAMP_P15/1
  PAY_OLSERVO_DAMP_P15/1 -> Out/1

== system typeAsimctrl_NB_upgrade_2016b/TypeA/Controller/BPcomb/OLSERVO_P16 ==
  In : Inport
  K1:VIS-OPTIC_PAY_OLSERVO_DAMP_P16 : LiveParts/LiveFilter  Tag=LiveFilter
      settings: AttributesFormatString=%<Tag>
  PAY_OLSERVO_DAMP_P16 : cstblocks/LTI System  sys=Filt('PAY_OLSERVO_DAMP_P16')  IC=[]
  Out : Outport
  wires:
  In/1 -> PAY_OLSERVO_DAMP_P16/1
  PAY_OLSERVO_DAMP_P16/1 -> Out/1

== system typeAsimctrl_NB_upgrade_2016b/TypeA/Controller/BPcomb/OLSERVO_P17 ==
  In : Inport
  K1:VIS-OPTIC_PAY_OLSERVO_DAMP_P17 : LiveParts/LiveFilter  Tag=LiveFilter
      settings: AttributesFormatString=%<Tag>
  PAY_OLSERVO_DAMP_P17 : cstblocks/LTI System  sys=Filt('PAY_OLSERVO_DAMP_P17')  IC=[]
  Out : Outport
  wires:
  In/1 -> PAY_OLSERVO_DAMP_P17/1
  PAY_OLSERVO_DAMP_P17/1 -> Out/1

== system typeAsimctrl_NB_upgrade_2016b/TypeA/Controller/BPcomb/OLSERVO_P18 ==
  In : Inport
  K1:VIS-OPTIC_PAY_OLSERVO_DAMP_P18 : LiveParts/LiveFilter  Tag=LiveFilter
      settings: AttributesFormatString=%<Tag>
  PAY_OLSERVO_DAMP_P18 : cstblocks/LTI System  sys=Filt('PAY_OLSERVO_DAMP_P18')  IC=[]
  Out : Outport
  wires:
  In/1 -> PAY_OLSERVO_DAMP_P18/1
  PAY_OLSERVO_DAMP_P18/1 -> Out/1

== system typeAsimctrl_NB_upgrade_2016b/TypeA/Controller/BPcomb/OLSERVO_P19 ==
  In : Inport
  K1:VIS-OPTIC_PAY_OLSERVO_DAMP_P19 : LiveParts/LiveFilter  Tag=LiveFilter
      settings: AttributesFormatString=%<Tag>
  PAY_OLSERVO_DAMP_P19 : cstblocks/LTI System  sys=Filt('PAY_OLSERVO_DAMP_P19')  IC=[]
  Out : Outport
  wires:
  In/1 -> PAY_OLSERVO_DAMP_P19/1
  PAY_OLSERVO_DAMP_P19/1 -> Out/1

== system typeAsimctrl_NB_upgrade_2016b/TypeA/Controller/BPcomb/OLSERVO_P21 ==
  In : Inport
  K1:VIS-OPTIC_PAY_OLSERVO_DAMP_P07 : LiveParts/LiveFilter  Tag=LiveFilter
      settings: AttributesFormatString=%<Tag>
  PAY_OLSERVO_DAMP_P21 : cstblocks/LTI System  sys=Filt('PAY_OLSERVO_DAMP_P21')  IC=[]
  Out : Outport
  wires:
  In/1 -> PAY_OLSERVO_DAMP_P21/1
  PAY_OLSERVO_DAMP_P21/1 -> Out/1

== system typeAsimctrl_NB_upgrade_2016b/TypeA/Controller/BPcomb/OLSERVO_P23 ==
  In : Inport
  K1:VIS-OPTIC_PAY_OLSERVO_DAMP_P23 : LiveParts/LiveFilter  Tag=LiveFilter
      settings: AttributesFormatString=%<Tag>
  PAY_OLSERVO_DAMP_P23 : cstblocks/LTI System  sys=Filt('PAY_OLSERVO_DAMP_P23')  IC=[]
  Out : Outport
  wires:
  In/1 -> PAY_OLSERVO_DAMP_P23/1
  PAY_OLSERVO_DAMP_P23/1 -> Out/1

== system typeAsimctrl_NB_upgrade_2016b/TypeA/Controller/BPcomb/OLSERVO_P24 ==
  In : Inport
  K1:VIS-OPTIC_PAY_OLSERVO_DAMP_P24 : LiveParts/LiveFilter  Tag=LiveFilter
      settings: AttributesFormatString=%<Tag>
  PAY_OLSERVO_DAMP_P24 : cstblocks/LTI System  sys=Filt('PAY_OLSERVO_DAMP_P24')  IC=[]
  Out : Outport
  wires:
  In/1 -> PAY_OLSERVO_DAMP_P24/1
  PAY_OLSERVO_DAMP_P24/1 -> Out/1

== system typeAsimctrl_NB_upgrade_2016b/TypeA/Controller/GASservo/Servo_GASBF ==
  In : Inport
  BF_DAMP_GAS : cstblocks/LTI System  sys=Filt('BF_DAMP_GAS')  IC=[]
  K1:VIS-OPTIC_BF_DAMP_GAS : LiveParts/LiveFilter  Tag=LiveFilter
      settings: AttributesFormatString=%<Tag>
  Out : Outport
  wires:
  In/1 -> BF_DAMP_GAS/1
  BF_DAMP_GAS/1 -> Out/1

== system typeAsimctrl_NB_upgrade_2016b/TypeA/Controller/GASservo/Servo_GASF0 ==
  In : Inport
  F0_DAMP_GAS : cstblocks/LTI System  sys=Filt('F0_DAMP_GAS')  IC=[]
  K1:VIS-OPTIC_F0_DAMP_GAS : LiveParts/LiveFilter  Tag=LiveFilter
      settings: AttributesFormatString=%<Tag>
  Out : Outport
  wires:
  In/1 -> F0_DAMP_GAS/1
  F0_DAMP_GAS/1 -> Out/1

== system typeAsimctrl_NB_upgrade_2016b/TypeA/Controller/GASservo/Servo_GASF1 ==
  In : Inport
  F1_DAMP_GAS : cstblocks/LTI System  sys=Filt('F1_DAMP_GAS')  IC=[]
  K1:VIS-OPTIC_F1_DAMP_GAS : LiveParts/LiveFilter  Tag=LiveFilter
      settings: AttributesFormatString=%<Tag>
  Out : Outport
  wires:
  In/1 -> F1_DAMP_GAS/1
  F1_DAMP_GAS/1 -> Out/1

== system typeAsimctrl_NB_upgrade_2016b/TypeA/Controller/GASservo/Servo_GASF2 ==
  In : Inport
  F2_DAMP_GAS : cstblocks/LTI System  sys=Filt('F2_DAMP_GAS')  IC=[]
  K1:VIS-OPTIC_F2_DAMP_GAS : LiveParts/LiveFilter  Tag=LiveFilter
      settings: AttributesFormatString=%<Tag>
  Out : Outport
  wires:
  In/1 -> F2_DAMP_GAS/1
  F2_DAMP_GAS/1 -> Out/1

== system typeAsimctrl_NB_upgrade_2016b/TypeA/Controller/GASservo/Servo_GASF3 ==
  In : Inport
  F3_DAMP_GAS : cstblocks/LTI System  sys=Filt('F3_DAMP_GAS')  IC=[]
  K1:VIS-OPTIC_F3_DAMP_GAS : LiveParts/LiveFilter  Tag=LiveFilter
      settings: AttributesFormatString=%<Tag>
  Out : Outport
  wires:
  In/1 -> F3_DAMP_GAS/1
  F3_DAMP_GAS/1 -> Out/1

== system typeAsimctrl_NB_upgrade_2016b/TypeA/Controller/IMservo/Damp_LIM ==
  In : Inport
  IM_PSDAMP_L : cstblocks/LTI System  sys=Filt('IM_PSDAMP_L')  IC=[]
  K1:VIS-OPTIC_IM_PSDAMP_L : LiveParts/LiveFilter  Tag=LiveFilter
      settings: AttributesFormatString=%<Tag>
  Out : Outport
  wires:
  In/1 -> IM_PSDAMP_L/1
  IM_PSDAMP_L/1 -> Out/1

== system typeAsimctrl_NB_upgrade_2016b/TypeA/Controller/IMservo/Damp_PIM ==
  In : Inport
  IM_PSDAMP_P : cstblocks/LTI System  sys=Filt('IM_PSDAMP_P')  IC=[]
  K1:VIS-OPTIC_IM_PSDAMP_P : LiveParts/LiveFilter  Tag=LiveFilter
      settings: AttributesFormatString=%<Tag>
  Out : Outport
  wires:
  In/1 -> IM_PSDAMP_P/1
  IM_PSDAMP_P/1 -> Out/1

== system typeAsimctrl_NB_upgrade_2016b/TypeA/Controller/IMservo/Damp_RIM ==
  In : Inport
  IM_PSDAMP_R : cstblocks/LTI System  sys=Filt('IM_PSDAMP_R')  IC=[]
  K1:VIS-OPTIC_IM_PSDAMP_R : LiveParts/LiveFilter  Tag=LiveFilter
      settings: AttributesFormatString=%<Tag>
  Out : Outport
  wires:
  In/1 -> IM_PSDAMP_R/1
  IM_PSDAMP_R/1 -> Out/1

== system typeAsimctrl_NB_upgrade_2016b/TypeA/Controller/IMservo/Damp_TIM ==
  In : Inport
  IM_PSDAMP_T : cstblocks/LTI System  sys=Filt('IM_PSDAMP_T')  IC=[]
  K1:VIS-OPTIC_IM_PSDAMP_T : LiveParts/LiveFilter  Tag=LiveFilter
      settings: AttributesFormatString=%<Tag>
  Out : Outport
  wires:
  In/1 -> IM_PSDAMP_T/1
  IM_PSDAMP_T/1 -> Out/1

== system typeAsimctrl_NB_upgrade_2016b/TypeA/Controller/IMservo/Damp_VIM ==
  In : Inport
  IM_PSDAMP_V : cstblocks/LTI System  sys=Filt('IM_PSDAMP_V')  IC=[]
  K1:VIS-OPTIC_IM_PSDAMP_V : LiveParts/LiveFilter  Tag=LiveFilter
      settings: AttributesFormatString=%<Tag>
  Out : Outport
  wires:
  In/1 -> IM_PSDAMP_V/1
  IM_PSDAMP_V/1 -> Out/1

== system typeAsimctrl_NB_upgrade_2016b/TypeA/Controller/IMservo/Damp_YIM ==
  In : Inport
  IM_PSDAMP_Y : cstblocks/LTI System  sys=Filt('IM_PSDAMP_Y')  IC=[]
  K1:VIS-OPTIC_IM_PSDAMP_Y : LiveParts/LiveFilter  Tag=LiveFilter
      settings: AttributesFormatString=%<Tag>
  Out : Outport
  wires:
  In/1 -> IM_PSDAMP_Y/1
  IM_PSDAMP_Y/1 -> Out/1

== system typeAsimctrl_NB_upgrade_2016b/TypeA/Controller/IMservo/IMLOCK_L ==
  In : Inport
  IM_LOCK_L : cstblocks/LTI System  sys=Filt('IM_LOCK_L')  IC=[]
  K1:VIS-OPTIC_IM_LOCK_L : LiveParts/LiveFilter  Tag=LiveFilter
      settings: AttributesFormatString=%<Tag>
  Out : Outport
  wires:
  In/1 -> IM_LOCK_L/1
  IM_LOCK_L/1 -> Out/1

== system typeAsimctrl_NB_upgrade_2016b/TypeA/Controller/IMservo/IMLOCK_P ==
  In : Inport
  IM_LOCK_P : cstblocks/LTI System  sys=Filt('IM_LOCK_P')  IC=[]
  K1:VIS-OPTIC_IM_LOCK_P : LiveParts/LiveFilter  Tag=LiveFilter
      settings: AttributesFormatString=%<Tag>
  Out : Outport
  wires:
  In/1 -> IM_LOCK_P/1
  IM_LOCK_P/1 -> Out/1

== system typeAsimctrl_NB_upgrade_2016b/TypeA/Controller/IMservo/IMLOCK_Y ==
  In : Inport
  IM_LOCK_Y : cstblocks/LTI System  sys=Filt('IM_LOCK_Y')  IC=[]
  K1:VIS-OPTIC_IM_LOCK_Y : LiveParts/LiveFilter  Tag=LiveFilter
      settings: AttributesFormatString=%<Tag>
  Out : Outport
  wires:
  In/1 -> IM_LOCK_Y/1
  IM_LOCK_Y/1 -> Out/1

== system typeAsimctrl_NB_upgrade_2016b/TypeA/Controller/IMservo/TMOLDamp_LIM ==
  In : Inport
  IM_TMOLDAMP_L : cstblocks/LTI System  sys=Filt('IM_TMOLDAMP_L')  IC=[]
  K1:VIS-OPTIC_IM_TMOLDAMP_L : LiveParts/LiveFilter  Tag=LiveFilter
      settings: AttributesFormatString=%<Tag>
  Out : Outport
  wires:
  In/1 -> IM_TMOLDAMP_L/1
  IM_TMOLDAMP_L/1 -> Out/1

== system typeAsimctrl_NB_upgrade_2016b/TypeA/Controller/IMservo/TMOLDamp_PIM ==
  In : Inport
  IM_TMOLDAMP_P : cstblocks/LTI System  sys=Filt('IM_TMOLDAMP_P')  IC=[]
  K1:VIS-OPTIC_IM_TMOLDAMP_P : LiveParts/LiveFilter  Tag=LiveFilter
      settings: AttributesFormatString=%<Tag>
  Out : Outport
  wires:
  In/1 -> IM_TMOLDAMP_P/1
  IM_TMOLDAMP_P/1 -> Out/1

== system typeAsimctrl_NB_upgrade_2016b/TypeA/Controller/IMservo/TMOLDamp_YIM ==
  In : Inport
  IM_TMOLDAMP_Y : cstblocks/LTI System  sys=Filt('IM_TMOLDAMP_Y')  IC=[]
  K1:VIS-OPTIC_IM_TMOLDAMP_Y : LiveParts/LiveFilter  Tag=LiveFilter
      settings: AttributesFormatString=%<Tag>
  Out : Outport
  wires:
  In/1 -> IM_TMOLDAMP_Y/1
  IM_TMOLDAMP_Y/1 -> Out/1

== system typeAsimctrl_NB_upgrade_2016b/TypeA/Controller/IPservo/Servo_LIP ==
  In : Inport
  IP_DAMP_L : cstblocks/LTI System  sys=Filt('IP_DAMP_L')  IC=[]
  K1:VIS-OPTIC_IP_DAMP_L : LiveParts/LiveFilter  Tag=LiveFilter
      settings: AttributesFormatString=%<Tag>
  Out : Outport
  wires:
  In/1 -> IP_DAMP_L/1
  IP_DAMP_L/1 -> Out/1

== system typeAsimctrl_NB_upgrade_2016b/TypeA/Controller/IPservo/Servo_TIP ==
  In : Inport
  IP_DAMP_T : cstblocks/LTI System  sys=Filt('IP_DAMP_T')  IC=[]
  K1:VIS-OPTIC_IP_DAMP_T : LiveParts/LiveFilter  Tag=LiveFilter
      settings: AttributesFormatString=%<Tag>
  Out : Outport
  wires:
  In/1 -> IP_DAMP_T/1
  IP_DAMP_T/1 -> Out/1

== system typeAsimctrl_NB_upgrade_2016b/TypeA/Controller/IPservo/Servo_YIP ==
  In : Inport
  IP_DAMP_Y : cstblocks/LTI System  sys=Filt('IP_DAMP_Y')  IC=[]
  K1:VIS-OPTIC_IP_DAMP_Y : LiveParts/LiveFilter  Tag=LiveFilter
      settings: AttributesFormatString=%<Tag>
  Out : Outport
  wires:
  In/1 -> IP_DAMP_Y/1
  IP_DAMP_Y/1 -> Out/1

== system typeAsimctrl_NB_upgrade_2016b/TypeA/Controller/MNservo/Damp_LMN ==
  In : Inport
  K1:VIS-OPTIC_MN_PSDAMP_L : LiveParts/LiveFilter  Tag=LiveFilter
      settings: AttributesFormatString=%<Tag>
  MN_PSDAMP_L : cstblocks/LTI System  sys=Filt('MN_PSDAMP_L')  IC=[]
  Out : Outport
  wires:
  In/1 -> MN_PSDAMP_L/1
  MN_PSDAMP_L/1 -> Out/1

== system typeAsimctrl_NB_upgrade_2016b/TypeA/Controller/MNservo/Damp_PMN ==
  In : Inport
  K1:VIS-OPTIC_MN_PSDAMP_P : LiveParts/LiveFilter  Tag=LiveFilter
      settings: AttributesFormatString=%<Tag>
  MN_PSDAMP_P : cstblocks/LTI System  sys=Filt('MN_PSDAMP_P')  IC=[]
  Out : Outport
  wires:
  In/1 -> MN_PSDAMP_P/1
  MN_PSDAMP_P/1 -> Out/1

== system typeAsimctrl_NB_upgrade_2016b/TypeA/Controller/MNservo/Damp_RMN ==
  In : Inport
  K1:VIS-OPTIC_MN_PSDAMP_R : LiveParts/LiveFilter  Tag=LiveFilter
      settings: AttributesFormatString=%<Tag>
  MN_PSDAMP_R : cstblocks/LTI System  sys=Filt('MN_PSDAMP_R')  IC=[]
  Out : Outport
  wires:
  In/1 -> MN_PSDAMP_R/1
  MN_PSDAMP_R/1 -> Out/1

== system typeAsimctrl_NB_upgrade_2016b/TypeA/Controller/MNservo/Damp_TMN ==
  In : Inport
  K1:VIS-OPTIC_MN_PSDAMP_T : LiveParts/LiveFilter  Tag=LiveFilter
      settings: AttributesFormatString=%<Tag>
  MN_PSDAMP_T : cstblocks/LTI System  sys=Filt('MN_PSDAMP_T')  IC=[]
  Out : Outport
  wires:
  In/1 -> MN_PSDAMP_T/1
  MN_PSDAMP_T/1 -> Out/1

== system typeAsimctrl_NB_upgrade_2016b/TypeA/Controller/MNservo/Damp_VMN ==
  In : Inport
  K1:VIS-OPTIC_MN_PSDAMP_V : LiveParts/LiveFilter  Tag=LiveFilter
      settings: AttributesFormatString=%<Tag>
  MN_PSDAMP_V : cstblocks/LTI System  sys=Filt('MN_PSDAMP_V')  IC=[]
  Out : Outport
  wires:
  In/1 -> MN_PSDAMP_V/1
  MN_PSDAMP_V/1 -> Out/1

== system typeAsimctrl_NB_upgrade_2016b/TypeA/Controller/MNservo/Damp_YMN ==
  In : Inport
  K1:VIS-OPTIC_MN_PSDAMP_Y : LiveParts/LiveFilter  Tag=LiveFilter
      settings: AttributesFormatString=%<Tag>
  MN_PSDAMP_Y : cstblocks/LTI System  sys=Filt('MN_PSDAMP_Y')  IC=[]
  Out : Outport
  wires:
  In/1 -> MN_PSDAMP_Y/1
  MN_PSDAMP_Y/1 -> Out/1

== system typeAsimctrl_NB_upgrade_2016b/TypeA/Controller/MNservo/MNLOCK_L ==
  In : Inport
  K1:VIS-OPTIC_MN_LOCK_L : LiveParts/LiveFilter  Tag=LiveFilter
      settings: AttributesFormatString=%<Tag>
  MN_LOCK_L : cstblocks/LTI System  sys=Filt('MN_LOCK_L')  IC=[]
  Out : Outport
  wires:
  In/1 -> MN_LOCK_L/1
  MN_LOCK_L/1 -> Out/1

== system typeAsimctrl_NB_upgrade_2016b/TypeA/Controller/MNservo/MNLOCK_P ==
  In : Inport
  K1:VIS-OPTIC_MN_LOCK_P : LiveParts/LiveFilter  Tag=LiveFilter
      settings: AttributesFormatString=%<Tag>
  MN_LOCK_P : cstblocks/LTI System  sys=Filt('MN_LOCK_P')  IC=[]
  Out : Outport
  wires:
  In/1 -> MN_LOCK_P/1
  MN_LOCK_P/1 -> Out/1

== system typeAsimctrl_NB_upgrade_2016b/TypeA/Controller/MNservo/MNLOCK_Y ==
  In : Inport
  K1:VIS-OPTIC_MN_LOCK_Y : LiveParts/LiveFilter  Tag=LiveFilter
      settings: AttributesFormatString=%<Tag>
  MN_LOCK_Y : cstblocks/LTI System  sys=Filt('MN_LOCK_Y')  IC=[]
  Out : Outport
  wires:
  In/1 -> MN_LOCK_Y/1
  MN_LOCK_Y/1 -> Out/1

== system typeAsimctrl_NB_upgrade_2016b/TypeA/Controller/MNservo/OLDamp_LMN ==
  In : Inport
  K1:VIS-OPTIC_MN_MNOLDAMP_L : LiveParts/LiveFilter  Tag=LiveFilter
      settings: AttributesFormatString=%<Tag>
  MN_MNOLDAMP_L : cstblocks/LTI System  sys=Filt('MN_MNOLDAMP_L')  IC=[]
  Out : Outport
  wires:
  In/1 -> MN_MNOLDAMP_L/1
  MN_MNOLDAMP_L/1 -> Out/1

== system typeAsimctrl_NB_upgrade_2016b/TypeA/Controller/MNservo/OLDamp_PMN ==
  In : Inport
  K1:VIS-OPTIC_MN_MNOLDAMP_P : LiveParts/LiveFilter  Tag=LiveFilter
      settings: AttributesFormatString=%<Tag>
  MN_MNOLDAMP_P : cstblocks/LTI System  sys=Filt('MN_MNOLDAMP_P')  IC=[]
  Out : Outport
  wires:
  In/1 -> MN_MNOLDAMP_P/1
  MN_MNOLDAMP_P/1 -> Out/1

== system typeAsimctrl_NB_upgrade_2016b/TypeA/Controller/MNservo/OLDamp_RMN ==
  In : Inport
  K1:VIS-OPTIC_MN_MNOLDAMP_R : LiveParts/LiveFilter  Tag=LiveFilter
      settings: AttributesFormatString=%<Tag>
  MN_MNOLDAMP_R : cstblocks/LTI System  sys=Filt('MN_MNOLDAMP_R')  IC=[]
  Out : Outport
  wires:
  In/1 -> MN_MNOLDAMP_R/1
  MN_MNOLDAMP_R/1 -> Out/1

== system typeAsimctrl_NB_upgrade_2016b/TypeA/Controller/MNservo/OLDamp_TMN ==
  In : Inport
  K1:VIS-OPTIC_MN_MNOLDAMP_T : LiveParts/LiveFilter  Tag=LiveFilter
      settings: AttributesFormatString=%<Tag>
  MN_MNOLDAMP_T : cstblocks/LTI System  sys=Filt('MN_MNOLDAMP_T')  IC=[]
  Out : Outport
  wires:
  In/1 -> MN_MNOLDAMP_T/1
  MN_MNOLDAMP_T/1 -> Out/1

== system typeAsimctrl_NB_upgrade_2016b/TypeA/Controller/MNservo/OLDamp_VMN ==
  In : Inport
  K1:VIS-OPTIC_MN_MNOLDAMP_V : LiveParts/LiveFilter  Tag=LiveFilter
      settings: AttributesFormatString=%<Tag>
  MN_MNOLDAMP_V : cstblocks/LTI System  sys=Filt('MN_MNOLDAMP_V')  IC=[]
  Out : Outport
  wires:
  In/1 -> MN_MNOLDAMP_V/1
  MN_MNOLDAMP_V/1 -> Out/1

== system typeAsimctrl_NB_upgrade_2016b/TypeA/Controller/MNservo/OLDamp_YMN ==
  In : Inport
  K1:VIS-OPTIC_MN_MNOLDAMP_Y : LiveParts/LiveFilter  Tag=LiveFilter
      settings: AttributesFormatString=%<Tag>
  MN_MNOLDAMP_Y : cstblocks/LTI System  sys=Filt('MN_MNOLDAMP_Y')  IC=[]
  Out : Outport
  wires:
  In/1 -> MN_MNOLDAMP_Y/1
  MN_MNOLDAMP_Y/1 -> Out/1

== system typeAsimctrl_NB_upgrade_2016b/TypeA/Controller/MNservo/TMOLDAMP_LMN ==
  In : Inport
  K1:VIS-OPTIC_MN_TMOLDAMP_L : LiveParts/LiveFilter  Tag=LiveFilter
      settings: AttributesFormatString=%<Tag>
  MN_TMOLDAMP_L : cstblocks/LTI System  sys=Filt('MN_TMOLDAMP_L')  IC=[]
  Out : Outport
  wires:
  In/1 -> MN_TMOLDAMP_L/1
  MN_TMOLDAMP_L/1 -> Out/1

== system typeAsimctrl_NB_upgrade_2016b/TypeA/Controller/MNservo/TMOLDAMP_PMN ==
  In : Inport
  K1:VIS-OPTIC_MN_TMOLDAMP_P : LiveParts/LiveFilter  Tag=LiveFilter
      settings: AttributesFormatString=%<Tag>
  MN_TMOLDAMP_P : cstblocks/LTI System  sys=Filt('MN_TMOLDAMP_P')  IC=[]
  Out : Outport
  wires:
  In/1 -> MN_TMOLDAMP_P/1
  MN_TMOLDAMP_P/1 -> Out/1
